simulink model "washing_machine"  (R2024b)
settings: Solver=VariableStepAuto  StartTime=0.0  StopTime=10.0  RelTol=1e-3
settings Model: Creator=Umesh Reddy K  LastModifiedBy=Umesh Reddy K

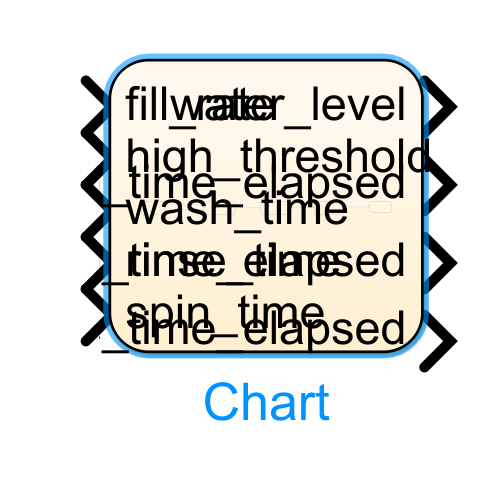
[thumbnail: Simulink's stored preview of the top-level diagram]
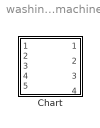
== system washing_machine ==
  Chart : Stateflow chart  TreatAsAtomicUnit=on

== stateflow chart washing_machine/Chart ==
  state Wash
    entry:
    disp('Washing clothes');
    wash_time_elapsed = wash_time_elapsed + 1;
    during:
    after(3, sec);
  state Rinse
    entry:
    disp('Rinsing clothes');
    rinse_time_elapsed = rinse_time_elapsed + 1;
    during:
    after(2, sec);
  state Spin
    entry:
    disp('Spinning clothes');
    spin_time_elapsed = spin_time_elapsed + 1;
    during:
    after(2, sec);
  state Done
    entry:
    disp('Washing cycle complete!');
  state Fill
    entry:
    disp('Filling water...');
    water_level = 0;
    water_level = water_level + fill_rate;
  (default) -> Fill
  Fill -> Wash : [water_level >= high_threshold]
  Spin -> Done : [spin_time_elapsed >= spin_time]
  Wash -> Rinse [order 2] : [wash_time_elapsed >= wash_time]
  Rinse -> Spin : [rinse_time_elapsed >= rinse_time]
  Wash -> Fill [order 1] : [water_level < high_threshold]
  data: fill_rate input; high_threshold input; wash_time input; rinse_time input; spin_time input; water_level output; wash_time_elapsed output; spin_time_elapsed output; rinse_time_elapsed output
